simulink model "AFI_sim_velest"  (R2022a)
settings: Solver=VariableStepAuto  StartTime=0.0  StopTime=84  MinStep=1e-4  RelTol=1e-3
undefined symbols (not defined in the file or in its folder): DiscIntNeverNeededParam
libraries: simulink x1
settings Model: Creator=bascetta  LastModifiedBy=bascetta
settings SolverCC: AlgebraicLoopSolver=TrustRegion
settings DataIOCC: SaveOutput=off  SignalLogging=off  DSMLogging=off  SaveTime=off  ReturnWorkspaceOutputs=off
settings DebuggingCC: UnconnectedInputMsg=warning  UnconnectedOutputMsg=warning  UnconnectedLineMsg=warning  SFMachineParentedDataDiag=warning

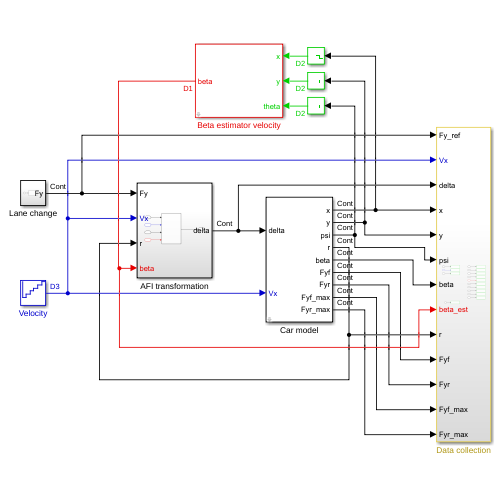
[thumbnail: Simulink's stored preview of the top-level diagram]
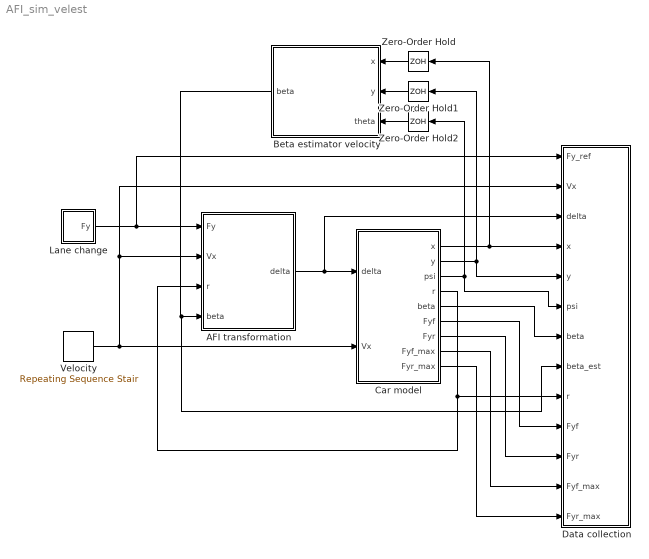
== system AFI_sim_velest ==
  AFI transformation : Subsystem
  Beta estimator velocity : Subsystem  mask{Kp=350, p=0.1, Ts=0.001, x0_vel=[0, 0, 0]}
      mask prompts: Kp "Proportional gain"; p "Point P position"; Ts "Sampling time"; x0_vel "Initial state (velocity)"
  Car model : Subsystem  mask{car_param=[0.1368, 0.1232, 1.9, 0.385, 50.13, 122.05, 0.029], initial_state=[0 0 0 0 0], tyre_model=0}
      mask prompts: car_param "Car parameters ([a b m mu Cf Cr Iz])"; initial_state "Initial state ([vy0 r0 psi0 x0 y0])"; tyre_model "Tyre model (0=Linear Model; 1='Fiala model; 2=Fiala without saturation)"
  Data collection : Subsystem
  Lane change : Subsystem
  Velocity : simulink/Sources/Repeating Sequence Stair  OutValues=[5:2:15].'  tsamp=14  OutMin=[]  OutMax=[]  OutDataTypeStr=double  OutputDataTypeScalingMode=double  OutDataType=fixdt(0,8)  ConRadixGroup=Best Precision: Vector-wise  OutScaling=2^-12
  Zero-Order Hold : ZeroOrderHold  SampleTime=0.01
  Zero-Order Hold1 : ZeroOrderHold  SampleTime=0.01
  Zero-Order Hold2 : ZeroOrderHold  SampleTime=0.01
  wires:
  AFI transformation/1(delta) -> Data collection/3(delta), Car model/1(delta)
  Car model/5(beta) -> Data collection/7(beta)
  Car model/4(r) -> AFI transformation/3(r), Data collection/9(r)
  Velocity/1 -> Car model/2(Vx), Data collection/2(Vx), AFI transformation/2(Vx)
  Lane change/1(Fy) -> Data collection/1(Fy_ref), AFI transformation/1(Fy)
  Car model/1(x) -> Zero-Order Hold/1, Data collection/4(x)
  Car model/2(y) -> Zero-Order Hold1/1, Data collection/5(y)
  Car model/3(psi) -> Zero-Order Hold2/1, Data collection/6(psi)
  Car model/6(Fyf) -> Data collection/10(Fyf)
  Car model/7(Fyr) -> Data collection/11(Fyr)
  Car model/9(Fyr_max) -> Data collection/13(Fyr_max)
  Car model/8(Fyf_max) -> Data collection/12(Fyf_max)
  Zero-Order Hold2/1 -> Beta estimator velocity/3(theta)
  Zero-Order Hold1/1 -> Beta estimator velocity/2(y)
  Zero-Order Hold/1 -> Beta estimator velocity/1(x)
  Beta estimator velocity/1(beta) -> Data collection/8(beta_est), AFI transformation/4(beta)

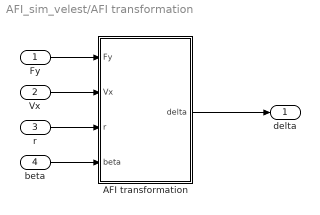
== system AFI_sim_velest/AFI transformation ==
  Fy : Inport
  Vx : Inport  Port=2
  r : Inport  Port=3
  beta : Inport  Port=4
  AFI transformation : Subsystem  mask{a=0.1368, Cf=50.13}
      mask DialogControl ParameterGroupVar Prompt: Car parameters
  delta : Outport
  wires:
  AFI transformation/1(delta) -> delta/1
  Vx/1 -> AFI transformation/2(Vx)
  beta/1 -> AFI transformation/4(beta)
  r/1 -> AFI transformation/3(r)
  Fy/1 -> AFI transformation/1(Fy)

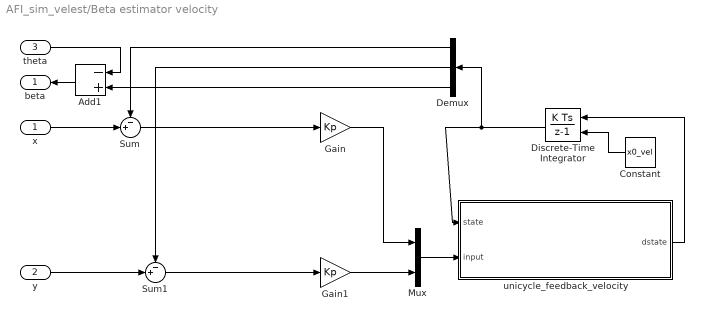
== system AFI_sim_velest/Beta estimator velocity ==
  x : Inport
  y : Inport  Port=2
  theta : Inport  Port=3
  Add1 : Sum  Inputs=-+
  Constant : Constant  Value=x0_vel
  Demux : Demux  Outputs=3
  Discrete-Time Integrator : DiscreteIntegrator  InitialConditionSource=external  SampleTime=Ts  ICPrevOutput=DiscIntNeverNeededParam  ICPrevScaledInput=DiscIntNeverNeededParam
  Gain : Gain  Gain=Kp
  Gain1 : Gain  Gain=Kp
  Mux : Mux  Inputs=2
  Sum : Sum  Inputs=-+|
  Sum1 : Sum  Inputs=-+|
  unicycle_feedback_velocity : MATLAB Function  TreatAsAtomicUnit=on
  beta : Outport  VectorParamsAs1DForOutWhenUnconnected=off
  wires:
  y/1 -> Sum1/2
  Demux/1 -> Sum/1
  Gain1/1 -> Mux/2
  Gain/1 -> Mux/1
  Mux/1 -> unicycle_feedback_velocity/2(input)
  Demux/2 -> Sum1/1
  x/1 -> Sum/2
  unicycle_feedback_velocity/1(dstate) -> Discrete-Time Integrator/1
  Discrete-Time Integrator/1 -> Demux/1, unicycle_feedback_velocity/1(state)
  Sum1/1 -> Gain1/1
  Sum/1 -> Gain/1
  Constant/1 -> Discrete-Time Integrator/2
  Demux/3 -> Add1/2
  theta/1 -> Add1/1
  Add1/1 -> beta/1

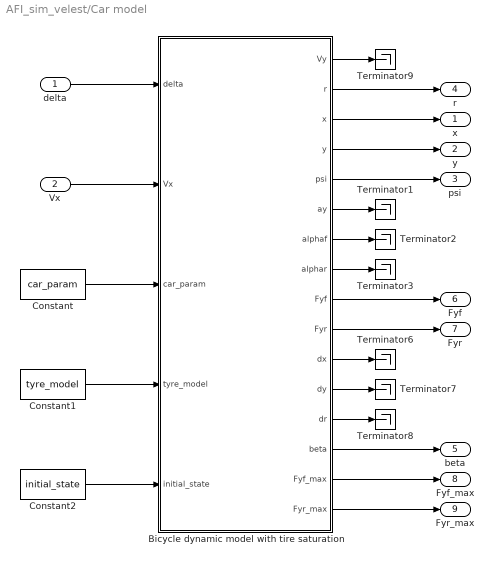
== system AFI_sim_velest/Car model ==
  delta : Inport
  Vx : Inport  Port=2
  Bicycle dynamic model with tire saturation : Subsystem
  Constant : Constant  Value=car_param
  Constant1 : Constant  Value=tyre_model
  Constant2 : Constant  Value=initial_state
  Terminator{1..3,6..9} (7 alike) : Terminator
  x : Outport
  y : Outport  Port=2
  psi : Outport  Port=3
  r : Outport  Port=4
  beta : Outport  Port=5
  Fyf : Outport  Port=6
  Fyr : Outport  Port=7
  Fyf_max : Outport  Port=8
  Fyr_max : Outport  Port=9
  wires:
  Constant1/1 -> Bicycle dynamic model with tire saturation/4(tyre_model)
  delta/1 -> Bicycle dynamic model with tire saturation/1(delta)
  Vx/1 -> Bicycle dynamic model with tire saturation/2(Vx)
  Constant2/1 -> Bicycle dynamic model with tire saturation/5("initial_state ")
  Bicycle dynamic model with tire saturation/3(x) -> x/1
  Bicycle dynamic model with tire saturation/4(y) -> y/1
  Constant/1 -> Bicycle dynamic model with tire saturation/3(car_param)
  Bicycle dynamic model with tire saturation/14(beta) -> beta/1
  Bicycle dynamic model with tire saturation/2(r) -> r/1
  Bicycle dynamic model with tire saturation/5(psi) -> psi/1
  Bicycle dynamic model with tire saturation/6(ay) -> Terminator1/1
  Bicycle dynamic model with tire saturation/7(alphaf) -> Terminator2/1
  Bicycle dynamic model with tire saturation/8(alphar) -> Terminator3/1
  Bicycle dynamic model with tire saturation/9(Fyf) -> Fyf/1
  Bicycle dynamic model with tire saturation/10(Fyr) -> Fyr/1
  Bicycle dynamic model with tire saturation/11(dx) -> Terminator6/1
  Bicycle dynamic model with tire saturation/12(dy) -> Terminator7/1
  Bicycle dynamic model with tire saturation/13(dr) -> Terminator8/1
  Bicycle dynamic model with tire saturation/1(Vy) -> Terminator9/1
  Bicycle dynamic model with tire saturation/15(Fyf_max) -> Fyf_max/1
  Bicycle dynamic model with tire saturation/16(Fyr_max) -> Fyr_max/1

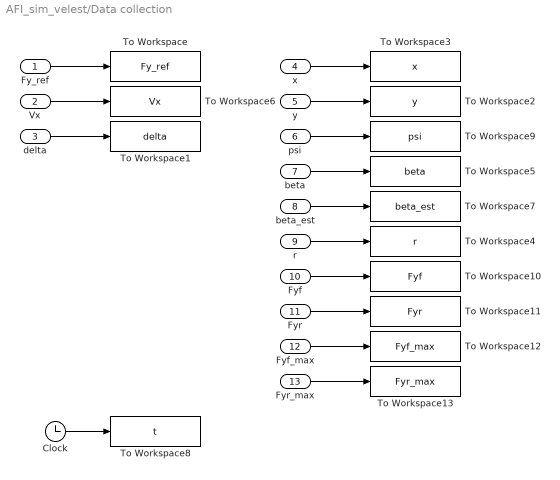
== system AFI_sim_velest/Data collection ==
  Fy_ref : Inport
  Vx : Inport  Port=2
  delta : Inport  Port=3
  x : Inport  Port=4
  y : Inport  Port=5
  psi : Inport  Port=6
  beta : Inport  Port=7
  beta_est : Inport  Port=8
  r : Inport  Port=9
  Fyf : Inport  Port=10
  Fyr : Inport  Port=11
  Fyf_max : Inport  Port=12
  Fyr_max : Inport  Port=13
  Clock : Clock
  To Workspace : ToWorkspace  VariableName=Fy_ref  SampleTime=0.01
  To Workspace1 : ToWorkspace  VariableName=delta  SampleTime=0.01
  To Workspace10 : ToWorkspace  VariableName=Fyf  SampleTime=0.01
  To Workspace11 : ToWorkspace  VariableName=Fyr  SampleTime=0.01
  To Workspace12 : ToWorkspace  VariableName=Fyf_max  SampleTime=0.01
  To Workspace13 : ToWorkspace  VariableName=Fyr_max  SampleTime=0.01
  To Workspace2 : ToWorkspace  VariableName=y  SampleTime=0.01
  To Workspace3 : ToWorkspace  VariableName=x  SampleTime=0.01
  To Workspace4 : ToWorkspace  VariableName=r  SampleTime=0.01
  To Workspace5 : ToWorkspace  VariableName=beta  SampleTime=0.01
  To Workspace6 : ToWorkspace  VariableName=Vx  SampleTime=0.01
  To Workspace7 : ToWorkspace  VariableName=beta_est  SampleTime=0.01
  To Workspace8 : ToWorkspace  VariableName=t  SampleTime=0.01
  To Workspace9 : ToWorkspace  VariableName=psi  SampleTime=0.01
  wires:
  beta/1 -> To Workspace5/1
  delta/1 -> To Workspace1/1
  Clock/1 -> To Workspace8/1
  r/1 -> To Workspace4/1
  x/1 -> To Workspace3/1
  Fy_ref/1 -> To Workspace/1
  Vx/1 -> To Workspace6/1
  y/1 -> To Workspace2/1
  psi/1 -> To Workspace9/1
  Fyf/1 -> To Workspace10/1
  Fyr/1 -> To Workspace11/1
  Fyf_max/1 -> To Workspace12/1
  Fyr_max/1 -> To Workspace13/1
  beta_est/1 -> To Workspace7/1

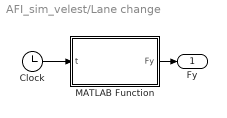
== system AFI_sim_velest/Lane change ==
  Clock : Clock
  MATLAB Function : MATLAB Function  TreatAsAtomicUnit=on
  Fy : Outport
  wires:
  Clock/1 -> MATLAB Function/1(t)
  MATLAB Function/1(Fy) -> Fy/1

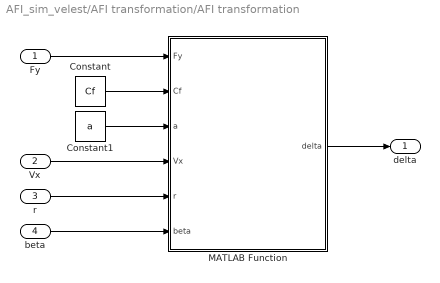
== system AFI_sim_velest/AFI transformation/AFI transformation ==
  Fy : Inport
  Vx : Inport  Port=2
  r : Inport  Port=3
  beta : Inport  Port=4
  Constant : Constant  Value=Cf
  Constant1 : Constant  Value=a
  MATLAB Function : MATLAB Function  TreatAsAtomicUnit=on
  delta : Outport
  wires:
  r/1 -> MATLAB Function/5(r)
  beta/1 -> MATLAB Function/6(beta)
  MATLAB Function/1(delta) -> delta/1
  Fy/1 -> MATLAB Function/1(Fy)
  Vx/1 -> MATLAB Function/4(Vx)
  Constant/1 -> MATLAB Function/2(Cf)
  Constant1/1 -> MATLAB Function/3(a)

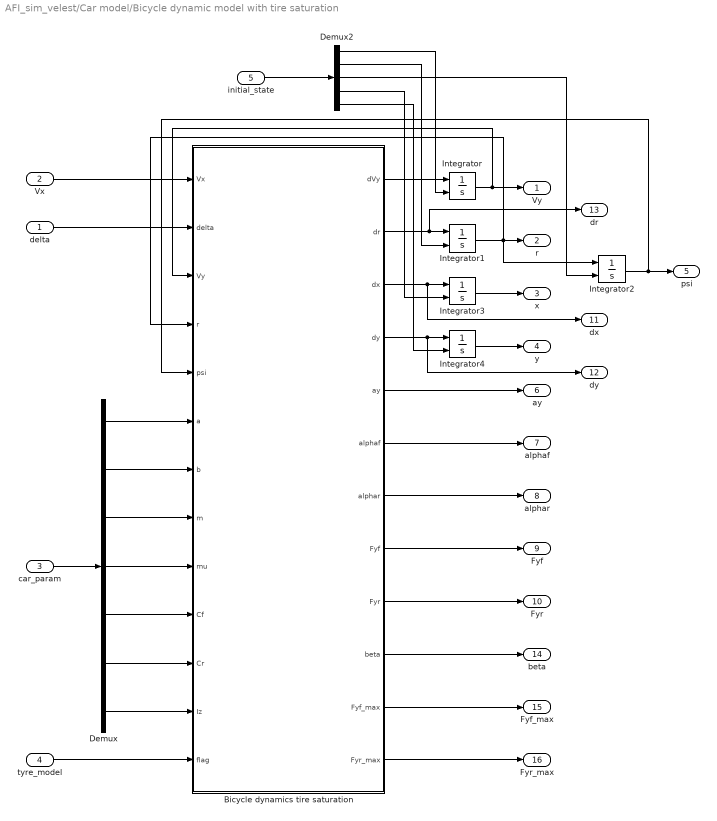
== system AFI_sim_velest/Car model/Bicycle dynamic model with tire saturation ==
  delta : Inport
  Vx : Inport  Port=2
  car_param : Inport  Port=3
  tyre_model : Inport  Port=4
  "initial_state " : Inport  Port=5
  Bicycle dynamics tire saturation : MATLAB Function  TreatAsAtomicUnit=on
  Demux : Demux  Outputs=7
  Demux2 : Demux  Outputs=5
  Integrator{,1..4} (5 alike) : Integrator  InitialConditionSource=external
  Vy : Outport
  r : Outport  Port=2
  x : Outport  Port=3
  y : Outport  Port=4
  psi : Outport  Port=5
  ay : Outport  Port=6
  alphaf : Outport  Port=7
  alphar : Outport  Port=8
  Fyf : Outport  Port=9
  Fyr : Outport  Port=10
  dx : Outport  Port=11
  dy : Outport  Port=12
  dr : Outport  Port=13
  beta : Outport  Port=14
  Fyf_max : Outport  Port=15
  Fyr_max : Outport  Port=16
  wires:
  Vx/1 -> Bicycle dynamics tire saturation/1(Vx)
  delta/1 -> Bicycle dynamics tire saturation/2(delta)
  Bicycle dynamics tire saturation/1(dVy) -> Integrator/1
  Bicycle dynamics tire saturation/2(dr) -> dr/1, Integrator1/1
  Integrator/1 -> Vy/1, Bicycle dynamics tire saturation/3(Vy)
  Integrator1/1 -> Bicycle dynamics tire saturation/4(r), r/1, Integrator2/1
  Bicycle dynamics tire saturation/5(ay) -> ay/1
  Bicycle dynamics tire saturation/6(alphaf) -> alphaf/1
  Bicycle dynamics tire saturation/7(alphar) -> alphar/1
  Bicycle dynamics tire saturation/8(Fyf) -> Fyf/1
  Bicycle dynamics tire saturation/9(Fyr) -> Fyr/1
  car_param/1 -> Demux/1
  Demux/1 -> Bicycle dynamics tire saturation/6(a)
  Demux/2 -> Bicycle dynamics tire saturation/7(b)
  Demux/3 -> Bicycle dynamics tire saturation/8(m)
  Demux/4 -> Bicycle dynamics tire saturation/9(mu)
  "initial_state "/1 -> Demux2/1
  Demux2/1 -> Integrator/2
  Demux2/2 -> Integrator1/2
  tyre_model/1 -> Bicycle dynamics tire saturation/13(flag)
  Demux/5 -> Bicycle dynamics tire saturation/10(Cf)
  Demux/6 -> Bicycle dynamics tire saturation/11(Cr)
  Demux/7 -> Bicycle dynamics tire saturation/12(Iz)
  Bicycle dynamics tire saturation/3(dx) -> dx/1, Integrator3/1
  Bicycle dynamics tire saturation/4(dy) -> dy/1, Integrator4/1
  Integrator3/1 -> x/1
  Integrator4/1 -> y/1
  Demux2/3 -> Integrator2/2
  Demux2/4 -> Integrator3/2
  Demux2/5 -> Integrator4/2
  Integrator2/1 -> Bicycle dynamics tire saturation/5(psi), psi/1
  Bicycle dynamics tire saturation/10(beta) -> beta/1
  Bicycle dynamics tire saturation/12(Fyr_max) -> Fyr_max/1
  Bicycle dynamics tire saturation/11(Fyf_max) -> Fyf_max/1

== matlab function AFI_sim_velest/Beta estimator velocity/unicycle_feedback_velocity ==
  data: state input size=3; dstate output size=3; input input size=2; p parameter size=1
function dstate = unicycle_feedback_velocity(state,input,p)

% State and input variables
x     = state(1);
y     = state(2);
gamma = state(3); % theta+beta

vxp   = input(1);
vyp   = input(2);


% Model equations
dstate = zeros(3,1);
dstate(1) = vxp*cos(gamma)^2+vyp*sin(gamma)*cos(gamma);
dstate(2) = vxp*sin(gamma)*cos(gamma)+vyp*sin(gamma)^2;
dstate(3) = (vyp*cos(gamma)-vxp*sin(gamma))/p;

== matlab function AFI_sim_velest/Lane change/MATLAB Function ==
  data: t input; Fy output
function Fy = lane_change(t)

if (mod(t,14)<=2)
    Fy = 0;
    return;
elseif (mod(t,14)<=4)
    Fy = -2;
    return;
elseif (mod(t,14)<=6)
    Fy = 2;
    return;
elseif (mod(t,14)<=8)
    Fy = 0;
    return;
elseif (mod(t,14)<=10)
    Fy = 2;
    return;
elseif (mod(t,14)<=12)
    Fy = -2;
    return;
else
    Fy = 0;
end

== matlab function AFI_sim_velest/Car model/Bicycle dynamic model with tire saturation/Bicycle dynamics tire saturation ==
  data: dVy output; Vx input; dr output; dx output; dy output; delta input; Vy input; r input; psi input; a input; b input; m input; mu input; Cf input; Cr input; Iz input; ay output; alphaf output; alphar output; Fyf output; Fyr output; flag input; beta output; Fyf_max output; Fyr_max output
function [dVy,dr,dx,dy,ay,alphaf,alphar,Fyf,Fyr,beta,Fyf_max,Fyr_max]  = bicycle_dynamics(Vx, delta, Vy, r, psi, a, b, m, mu, Cf, Cr, Iz, flag)

Fzf = m*9.81*b/(a+b);
Fzr = m*9.81*a/(a+b);

if (abs(Vx)<=0.01)
    alphaf = 0;
    alphar = 0;
else
    alphaf = atan((Vy+a*r)/Vx)-delta;
    alphar = atan((Vy-b*r)/Vx);
end

zf = tan(alphaf);
zr = tan(alphar);

zf_sl = 3*mu*Fzf/Cf;
zr_sl = 3*mu*Fzr/Cr;

switch flag
    case 0 % Linear tyre model
        Fyf = -Cf*alphaf;
        Fyr = -Cr*alphar;
    case 1 % Fiala model with saturation
        if (abs(zf)<zf_sl)
            Fyf = Cf*zf*(-1+abs(zf)/zf_sl-zf^2/(3*zf_sl^2));
        else
            Fyf = -mu*Fzf*sign(alphaf);
        end
        if (abs(zr)<zr_sl)
            Fyr = Cr*zr*(-1+abs(zr)/zr_sl-zr^2/(3*zr_sl^2));
        else
            Fyr = -mu*Fzr*sign(alphar);
        end
    case 2 % Fiala model without saturation
        Fyf = Cf*zf*(-1+abs(zf)/zf_sl-zf^2/(3*zf_sl^2));
        Fyr = Cr*zr*(-1+abs(zr)/zr_sl-zr^2/(3*zr_sl^2));
    otherwise
        Fyf = 0;
        Fyr = 0;
end

% Dynamic equations
dr  = (a*Fyf*cos(delta)-b*Fyr)/Iz;
dVy = (Fyf*cos(delta)+Fyr)/m-r*Vx;
ay  = dVy+r*Vx;

% Kinematic equations
R_psi = [cos(psi), -sin(psi); sin(psi), cos(psi)];
dx  = R_psi(1,1:2)*[Vx; Vy];
dy  = R_psi(2,1:2)*[Vx; Vy];

% Sideslip
if (abs(Vx)<=0.01)
    beta = 0;
else
    beta = atan2(Vy,Vx);
end

% Wheel forces
Fyf_max = mu*Fzf;
Fyr_max = mu*Fzr;

== matlab function AFI_sim_velest/AFI transformation/AFI transformation/MATLAB Function ==
  data: Fy input; delta output; Cf input; a input; Vx input; r input; beta input
function delta = AFI_transformation(Fy,Cf,a,Vx,r,beta)

delta = 1/Cf*Fy+[1, a/Vx]*[beta; r];
